simulink model "computedTorqueControl"  (Simulink 8.4)
settings: Solver=FixedStepDiscrete  StartTime=0.0  StopTime=Inf  FixedStep=Ts  RelTol=1e-3
InitFcn:
  | init_computedTorqueControl;
values from neighbouring files (symbols this model uses):
  ampl_and_freq = [ 20 ... (first row only)    [init_computedTorqueControl.m]    (also in init_computedTorqueControlV2.m)
  Kd = 2*sqrt(Kp)    [init_computedTorqueControl.m]    (also in init_computedTorqueControlV2.m)
  Kp = 70*diag( ones(1,ROBOT_DOF)  )    [init_computedTorqueControl.m]    (also in init_computedTorqueControlV2.m = 250*diag( ones(1,ROBOT_DOF)  ))
  ROBOT_DOF = 1    [init_computedTorqueControl.m]    (also in init_computedTorqueControlV2.m)
libraries: WBCLibrary x7
settings Model: Creator=daniele  LastModifiedBy=pucci
settings OptimizationCC: ExpressionDepthLimit=128
settings DebuggingCC: UnderspecifiedInitializationDetection=Simplified  MergeDetectMultiDrivingBlocksExec=error  MultiTaskDSMMsg=warning  MultiTaskCondExecSysMsg=none  FcnCallInpInsideContextMsg=EnableAllAsError  StateNameClashWarn=none  StrictBusMsg=ErrorOnBusTreatedAsVector
settings RTWCC: IncludeERTFirstTime=on
settings GRTTargetCC: CombineOutputUpdateFcns=on  GRTInterface=off

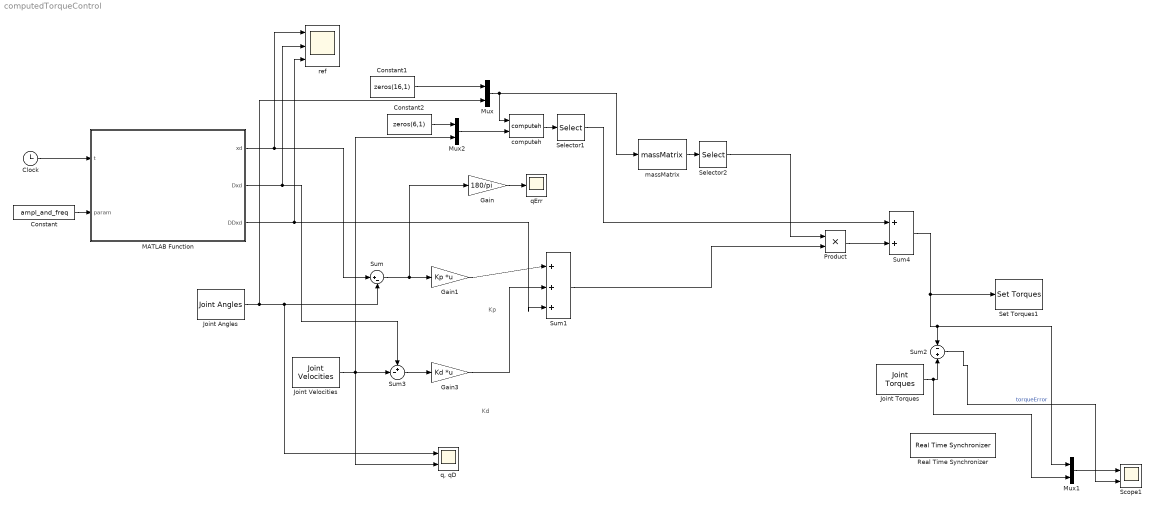
== system computedTorqueControl ==
  note: Kd
  note: Kp
  Clock : Clock
  Constant : Constant  Value=ampl_and_freq
  Constant1 : Constant  Value=zeros(16,1)
  Constant2 : Constant  Value=zeros(6,1)
  Gain : Gain  Gain=180/pi
  Gain1 : Gain  Gain=Kp  Multiplication=Matrix(K*u)
  Gain3 : Gain  Gain=Kd  Multiplication=Matrix(K*u)
  Joint Angles : WBCLibrary/wholeBodyStates/Joint Angles  robotName=robotName  localName=localName
  Joint Torques : WBCLibrary/wholeBodyStates/Joint Torques  robotName=robotName  localName=localName
  Joint Velocities : WBCLibrary/wholeBodyStates/Joint Velocities  robotName=robotName  localName=localName
  MATLAB Function : MATLAB Function  TreatAsAtomicUnit=on
  Mux : Mux  Inputs=2
  Mux1 : Mux  Inputs=2
  Mux2 : Mux  Inputs=2
  Product : Product
  Real Time Synchronizer : WBCLibrary/Utilities/Real Time Synchronizer  Priority=-10  threadPeriod=Ts
  Scope1 : Scope  NumInputPorts=2
      settings: YMin=-5~-5  YMax=5~5
  Selector1 : Selector  InputPortWidth=ROBOT_DOF+6  Indices=[7:ROBOT_DOF+6]
  Selector2 : Selector  NumberOfDimensions=2  InputPortWidth=ROBOT_DOF+6  IndexOptions=Index vector (dialog),Index vector (dialog)  Indices=[7:ROBOT_DOF+6],[7:ROBOT_DOF+6]  OutputSizes=1,1
  Set Torques1 : WBCLibrary/wholeBodyActuators/Set Torques  val=6  robotName=robotName  localName=localName
  Sum : Sum  Inputs=|+-
  Sum1 : Sum  Inputs=|+++
  Sum2 : Sum  Inputs=-|+
  Sum3 : Sum  Inputs=+-|
  Sum4 : Sum
  computeh : WBCLibrary/wholeBodyModel/Dynamics/computeh  val=7  robotname=robotName  localname=localName
  massMatrix : WBCLibrary/wholeBodyModel/Dynamics/massMatrix  val=8  robotname=robotName  localname=localName
  "q, qD" : Scope  NumInputPorts=2
      settings: YMin=-5~-5  YMax=5~5
  qErr : Scope
      settings: SaveName=ScopeData2
  ref : Scope  NumInputPorts=3
      settings: YMin=-5~-5~-5  YMax=5~5~5  SaveName=ScopeData3
  wires:
  Clock/1 -> MATLAB Function/1(t)
  Constant/1 -> MATLAB Function/2(param)
  Joint Angles/1 -> "q, qD"/1, Sum/2, Mux/2
  MATLAB Function/1(xd) -> ref/1, Sum/1
  Gain1/1 -> Sum1/1
  Mux2/1 -> computeh/2
  computeh/1 -> Selector1/1
  Mux/1 -> computeh/1, massMatrix/1
  Constant1/1 -> Mux/1
  Joint Torques/1 -> Mux1/2, Sum2/2
  Sum2/1 -> Scope1/2  "torqueError"
  Mux1/1 -> Scope1/1
  Sum/1 -> Gain1/1, Gain/1
  Sum3/1 -> Gain3/1
  MATLAB Function/2(Dxd) -> ref/2, Sum3/1
  Gain3/1 -> Sum1/2
  Gain/1 -> qErr/1
  Selector1/1 -> Sum4/1
  Sum4/1 -> Sum2/1, Mux1/1, Set Torques1/1
  MATLAB Function/3(DDxd) -> ref/3, Sum1/3
  massMatrix/1 -> Selector2/1
  Product/1 -> Sum4/2
  Selector2/1 -> Product/1
  Sum1/1 -> Product/2
  Joint Velocities/1 -> Sum3/2, "q, qD"/2, Mux2/2
  Constant2/1 -> Mux2/1

== matlab function MATLAB Function ==
  data: t input double; xd output double; param input double; Dxd output double; DDxd output double
function [xd,Dxd,DDxd] = fcn(t,param)
%#codegen

xd =  param(1)*sin(param(2)*t);

Dxd =  param(1)*param(2)*cos(param(2)*t);

DDxd = -param(1)*param(2)^2*sin(param(2)*t);
